simulink model "pendulum_project"  (Simulink 4.00)
settings: Solver=ode45  SolverMode=SingleTasking  StartTime=0.0  StopTime=100  RelTol=1e-4  AbsTol=1e-7
libraries: simulink3 x1
settings Model: LimitDataPoints=off  BlockReductionOpt=off

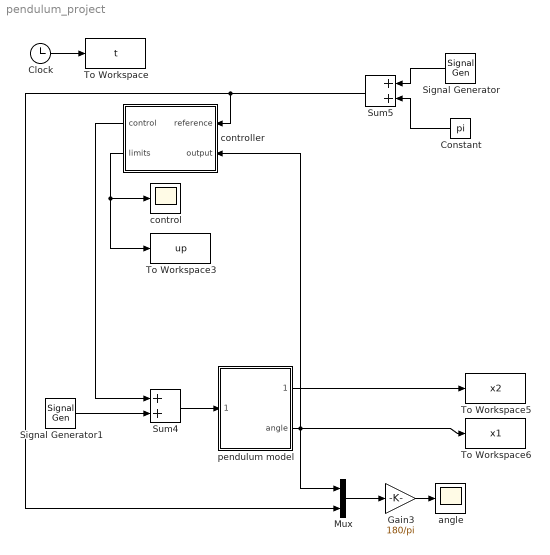
== system pendulum_project ==
  Clock : Clock
      settings: DisplayTime=off  Decimation=10
  Constant : Constant  Orientation=left  Value=pi
  Gain3 : Gain  Gain=180/pi  Multiplication=Element-wise(K.*u)  SaturateOnIntegerOverflow=on
  Mux : Mux  Inputs=2
  Signal Generator : SignalGenerator  Orientation=left  WaveForm=square  Amplitude=12*pi/180  Frequency=.1  Units=Hertz
  Signal Generator1 : SignalGenerator  WaveForm=square  Amplitude=.1  Frequency=.04  Units=Hertz
  Sum4 : Sum  Inputs=++  SaturateOnIntegerOverflow=on
  Sum5 : Sum  Orientation=left  Inputs=++  SaturateOnIntegerOverflow=on
  To Workspace : ToWorkspace  VariableName=t  SampleTime=.01  SaveFormat=Array
  To Workspace3 : ToWorkspace  VariableName=up  SampleTime=.01  SaveFormat=Array
  To Workspace5 : ToWorkspace  VariableName=x2  SampleTime=.01  SaveFormat=Array
  To Workspace6 : ToWorkspace  VariableName=x1  SampleTime=.01  SaveFormat=Array
  angle : Scope
      settings: TickLabels=on  TimeRange=100  YMin=165  YMax=195  SaveToWorkspace=off  SaveName=ScopeData  DataFormat=Array  MaxDataPoints=10000
  control : Scope
      settings: TickLabels=on  TimeRange=100  YMin=-2  YMax=2  SaveToWorkspace=off  SaveName=ScopeData  DataFormat=Array  MaxDataPoints=10000
  controller : Subsystem  Orientation=left
      settings: RTWFcnNameOpts=Auto  RTWFileNameOpts=Auto
  pendulum model : Subsystem  mask{mass=.275, length=0.5, friction=.01, Tmax=.5, quant=.1, stiction=.01, IC=0}
      mask prompts: friction "friction coeff"; Tmax "Max Torque"; quant "quantization (deg)"; stiction "stiction dead-zone (rad/s)"; IC "Initial condition (deg, 0 velocity)"
      settings: RTWFcnNameOpts=Auto  RTWFileNameOpts=Auto
  wires:
  pendulum model/1(velocity) -> To Workspace5/1
  Sum4/1 -> pendulum model/1(control)
  Signal Generator1/1 -> Sum4/2
  Gain3/1 -> angle/1
  Clock/1 -> To Workspace/1
  controller/1(control) -> Sum4/1
  controller/2(limits) -> control/1, To Workspace3/1
  pendulum model/2(angle) -> To Workspace6/1, Mux/1, controller/2(output)
  Signal Generator/1 -> Sum5/1
  Constant/1 -> Sum5/2
  Sum5/1 -> controller/1(reference), Mux/2
  Mux/1 -> Gain3/1

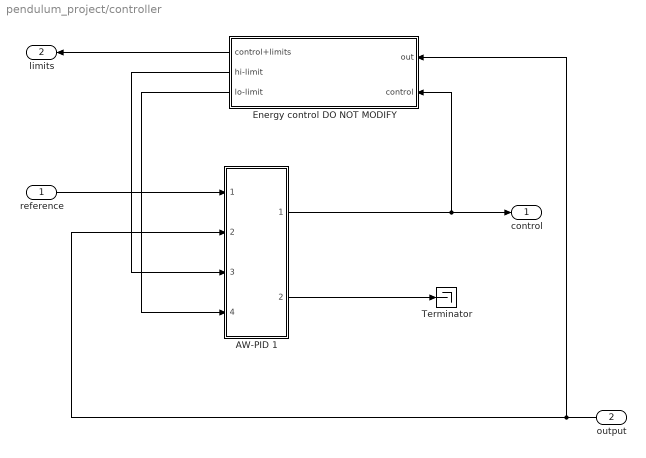
== system pendulum_project/controller ==
  reference : Inport  Port=1  LatchInput=off
  output : Inport  Orientation=left  Port=2  LatchInput=off
  AW-PID 1 : Subsystem  mask(Anti-windup PID ){kpid=[11, 30, 1.5], TCD=.01, TF=0, DT=.01, ipole=0, t_pref=[0.05, 0.4]}
      mask prompts: kpid "PID parameters [kp,ki,kd]"; TCD "Pseudo-derivative filter time constant"; TF "Error lowpass filter Time constant"; DT "Sampling Time"; ipole "Approx. Integrator pole"; t_pref "Reference prefilter [num,den] time constants"
      mask help: Discrete PID with Anti-windup, prefilter, and lowpass filter
      mask init:
      | t_z=t_pref(1);t_p=t_pref(2);
      settings: RTWFcnNameOpts=Auto  RTWFileNameOpts=Auto
      mask Display: disp('AW-PID\n+filter+init')
  Energy control DO NOT MODIFY : Subsystem  Orientation=left
      settings: RTWFcnNameOpts=Auto  RTWFileNameOpts=Auto
  Terminator : Terminator
  control : Outport  Port=1  InitialOutput=0
  limits : Outport  Orientation=left  Port=2  InitialOutput=0
  wires:
  Energy control DO NOT MODIFY/1(control+limits) -> limits/1
  output/1 -> Energy control DO NOT MODIFY/1(out), AW-PID 1/2(System Output)
  AW-PID 1/2(sat_indicator) -> Terminator/1
  AW-PID 1/1(Input to system) -> control/1, Energy control DO NOT MODIFY/2(control)
  reference/1 -> AW-PID 1/1(Set point)
  Energy control DO NOT MODIFY/2(hi-limit) -> AW-PID 1/3(input constraint hi)
  Energy control DO NOT MODIFY/3(lo-limit) -> AW-PID 1/4(input constraint lo)

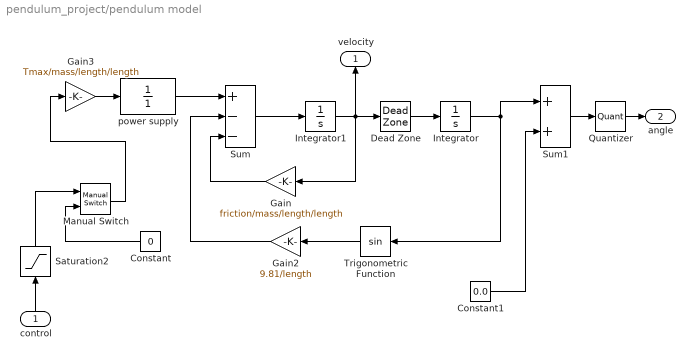
== system pendulum_project/pendulum model ==
  control : Inport  Orientation=up  Port=1  LatchInput=off
  Constant : Constant  Orientation=left  Value=0
  Constant1 : Constant  Value=0.0
  Dead Zone : DeadZone  LowerValue=-stiction  UpperValue=stiction  SaturateOnIntegerOverflow=on  LinearizeAsGain=on
  Gain : Gain  Orientation=left  Gain=friction/mass/length/length  Multiplication=Element-wise(K.*u)  SaturateOnIntegerOverflow=on
  Gain2 : Gain  Orientation=left  Gain=9.81/length  Multiplication=Element-wise(K.*u)  SaturateOnIntegerOverflow=on
  Gain3 : Gain  Gain=Tmax/mass/length/length  Multiplication=Element-wise(K.*u)  SaturateOnIntegerOverflow=on
  Integrator : Integrator  ExternalReset=none  InitialConditionSource=internal  InitialCondition=IC*pi/180  LimitOutput=off  UpperSaturationLimit=inf  LowerSaturationLimit=-inf  ShowSaturationPort=off  ShowStatePort=off  AbsoluteTolerance=auto
  Integrator1 : Integrator  ExternalReset=none  InitialConditionSource=internal  InitialCondition=0  LimitOutput=off  UpperSaturationLimit=inf  LowerSaturationLimit=-inf  ShowSaturationPort=off  ShowStatePort=off  AbsoluteTolerance=auto
  Manual Switch : simulink3/Nonlinear/Manual Switch  sw=1  action=0
  Quantizer : Quantizer  QuantizationInterval=quant*pi/180  LinearizeAsGain=on
  Saturation2 : Saturate  Orientation=up  UpperLimit=1  LowerLimit=-1  LinearizeAsGain=on
  Sum : Sum  Inputs=+--  SaturateOnIntegerOverflow=on
  Sum1 : Sum  Inputs=++  SaturateOnIntegerOverflow=on
  Trigonometric Function : Trigonometry  Orientation=left  Operator=sin  OutputSignalType=auto
  power supply : TransferFcn  Numerator=1  Denominator=1  AbsoluteTolerance=auto  Realization=auto
  velocity : Outport  Orientation=up  Port=1  InitialOutput=0
  angle : Outport  Port=2  InitialOutput=0
  wires:
  Sum/1 -> Integrator1/1
  Integrator1/1 -> Gain/1, velocity/1, Dead Zone/1
  Gain/1 -> Sum/3
  Dead Zone/1 -> Integrator/1
  Integrator/1 -> Sum1/1, Trigonometric Function/1
  Trigonometric Function/1 -> Gain2/1
  Gain2/1 -> Sum/2
  Gain3/1 -> power supply/1
  power supply/1 -> Sum/1
  control/1 -> Saturation2/1
  Manual Switch/1 -> Gain3/1
  Constant/1 -> Manual Switch/2
  Constant1/1 -> Sum1/2
  Sum1/1 -> Quantizer/1
  Quantizer/1 -> angle/1
  Saturation2/1 -> Manual Switch/1

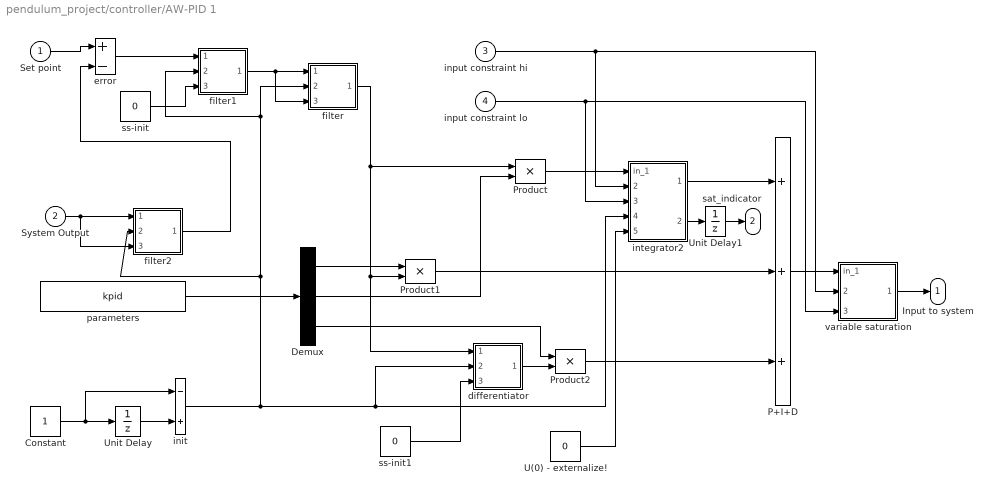
== system pendulum_project/controller/AW-PID 1 ==
  Set point : Inport  Port=1  LatchInput=off
  System Output : Inport  Port=2  LatchInput=off
  input constraint hi : Inport  Port=3  LatchInput=off
  input constraint lo : Inport  Port=4  LatchInput=off
  Constant : Constant  Value=1
  Demux : Demux  Outputs=3  BusSelectionMode=off
  P+I+D : Sum  Inputs=+++  SaturateOnIntegerOverflow=on
  Product : Product  Inputs=2  Multiplication=Element-wise(.*)  SaturateOnIntegerOverflow=on
  Product1 : Product  Inputs=2  Multiplication=Element-wise(.*)  SaturateOnIntegerOverflow=on
  Product2 : Product  Inputs=2  Multiplication=Element-wise(.*)  SaturateOnIntegerOverflow=on
  U(0) - externalize! : Constant  Value=0
  Unit Delay : UnitDelay  X0=0  SampleTime=DT
      settings: RTWStateStorageClass=Auto
  Unit Delay1 : UnitDelay  X0=0  SampleTime=DT
      settings: RTWStateStorageClass=Auto
  differentiator : Subsystem  mask(Approx. Differentator){DT=DT, TC=TCD}
      mask prompts: DT "sampling time"; TC "Time constant"
      settings: RTWFcnNameOpts=Auto  RTWFileNameOpts=Auto
  error : Sum  Inputs=+-  SaturateOnIntegerOverflow=on
  filter : Subsystem  mask(Lead-Lag Filter){DT=DT, TC=TF, TZ=0}
      mask prompts: DT "sampling time"; TC "Pole Time constant"; TZ "Zero Time Constant"
      settings: RTWFcnNameOpts=Auto  RTWFileNameOpts=Auto
  filter1 : Subsystem  mask(Lead-Lag Filter){DT=DT, TC=t_p, TZ=t_z}
      mask prompts: DT "sampling time"; TC "Pole Time constant"; TZ "Zero Time Constant"
      settings: RTWFcnNameOpts=Auto  RTWFileNameOpts=Auto
  filter2 : Subsystem  mask(Lead-Lag Filter){DT=DT, TC=t_z, TZ=t_p}
      mask prompts: DT "sampling time"; TC "Pole Time constant"; TZ "Zero Time Constant"
      settings: RTWFcnNameOpts=Auto  RTWFileNameOpts=Auto
  init : Sum  Inputs=-+  SaturateOnIntegerOverflow=on
  integrator2 : Subsystem  mask(Anti windup intgrator){DT=DT, pole=ipole}
      mask prompts: DT "sampling time"
      mask help: Integral with anti-windup
      settings: RTWFcnNameOpts=Auto  RTWFileNameOpts=Auto
  parameters : Constant  Value=kpid
  ss-init : Constant  Value=0
  ss-init1 : Constant  Value=0
  variable saturation : Subsystem  mask(Anti windup intgrator){DT=DT}
      mask prompts: DT "sampling time"
      mask help: Integral with anti-windup
      settings: RTWFcnNameOpts=Auto  RTWFileNameOpts=Auto
      mask Display: disp('DT-I-AW')
  Input to system : Outport  Port=1  InitialOutput=0
  sat_indicator : Outport  Port=2  InitialOutput=0
  wires:
  input constraint hi/1 -> variable saturation/2(umax), integrator2/2(umax)
  input constraint lo/1 -> variable saturation/3(umin), integrator2/3(umin)
  variable saturation/1(out_1) -> Input to system/1
  filter2/1(out_1) -> error/2
  System Output/1 -> filter2/1(in_1), filter2/3(init val)
  filter1/1(out_1) -> filter/1(in_1), filter/3(init val)
  Product2/1 -> P+I+D/3
  Demux/2 -> Product/2
  Demux/1 -> Product1/1
  Product/1 -> integrator2/1(in_1)
  P+I+D/1 -> variable saturation/1(in_1)
  integrator2/1(out_1) -> P+I+D/1
  error/1 -> filter1/1(in_1)
  parameters/1 -> Demux/1
  Set point/1 -> error/1
  Product1/1 -> P+I+D/2
  Demux/3 -> Product2/1
  differentiator/1(out_1) -> Product2/2
  filter/1(out_1) -> Product/1, Product1/2, differentiator/1(in_1)
  Constant/1 -> Unit Delay/1, init/1
  Unit Delay/1 -> init/2
  init/1 -> differentiator/2(init flag), integrator2/4(init flag), filter2/2(init flag), filter/2(init flag), filter1/2(init flag)
  integrator2/2(out_2) -> Unit Delay1/1
  U(0) - externalize!/1 -> integrator2/5(init val)
  ss-init/1 -> filter1/3(init val)
  ss-init1/1 -> differentiator/3(init val)
  Unit Delay1/1 -> sat_indicator/1

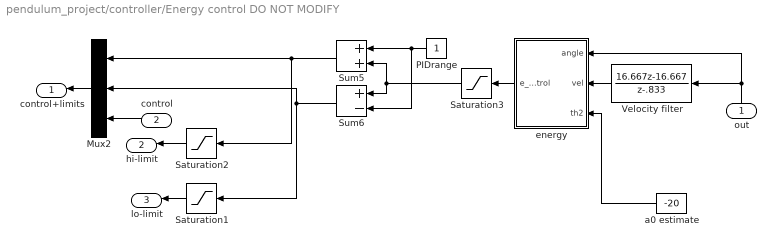
== system pendulum_project/controller/Energy control DO NOT MODIFY ==
  out : Inport  Orientation=up  Port=1  LatchInput=off
  control : Inport  Orientation=left  Port=2  LatchInput=off
  Mux2 : Mux  Orientation=left  Inputs=3
      settings: DisplayOption=none
  PIDrange : Constant  Orientation=left  Value=1
  Saturation1 : Saturate  Orientation=left  UpperLimit=1  LowerLimit=-1  LinearizeAsGain=on
  Saturation2 : Saturate  Orientation=left  UpperLimit=1  LowerLimit=-1  LinearizeAsGain=on
  Saturation3 : Saturate  Orientation=left  UpperLimit=1  LowerLimit=-1  LinearizeAsGain=on
  Sum5 : Sum  Orientation=left  Inputs=++  SaturateOnIntegerOverflow=on
  Sum6 : Sum  Orientation=left  Inputs=+-  SaturateOnIntegerOverflow=on
  Velocity filter : DiscreteTransferFcn  Orientation=left  Numerator="[16.667  -16.667]"  Denominator=[1 -.833]  SampleTime=.01  Realization=auto
      settings: RTWStateStorageClass=Auto
  a0 estimate : Constant  Orientation=left  Value=-20
  energy : Subsystem  Orientation=left
      settings: RTWFcnNameOpts=Auto  RTWFileNameOpts=Auto
  control+limits : Outport  Orientation=left  Port=1
  hi-limit : Outport  Orientation=left  Port=2
  lo-limit : Outport  Orientation=left  Port=3
  wires:
  Sum5/1 -> Mux2/1, Saturation2/1
  Sum6/1 -> Mux2/2, Saturation1/1
  energy/1(e_control) -> Saturation3/1
  Velocity filter/1 -> energy/2(vel)
  PIDrange/1 -> Sum5/1, Sum6/2
  Saturation3/1 -> Sum6/1, Sum5/2
  out/1 -> Velocity filter/1, energy/1(angle)
  a0 estimate/1 -> energy/3(th2)
  control/1 -> Mux2/3
  Mux2/1 -> control+limits/1
  Saturation2/1 -> hi-limit/1
  Saturation1/1 -> lo-limit/1

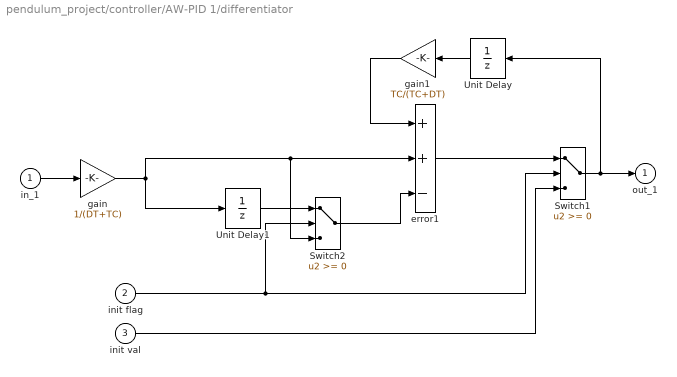
== system pendulum_project/controller/AW-PID 1/differentiator ==
  in_1 : Inport  Port=1  LatchInput=off
  init flag : Inport  Port=2  LatchInput=off
  init val : Inport  Port=3  LatchInput=off
  Switch1 : Switch  Threshold=0
  Switch2 : Switch  Threshold=0
  Unit Delay : UnitDelay  Orientation=left  X0=0  SampleTime=DT
      settings: RTWStateStorageClass=Auto
  Unit Delay1 : UnitDelay  X0=0  SampleTime=DT
      settings: RTWStateStorageClass=Auto
  error1 : Sum  Inputs=++-  SaturateOnIntegerOverflow=on
  gain : Gain  Gain=1/(DT+TC)  Multiplication=Element-wise(K.*u)  SaturateOnIntegerOverflow=on
  gain1 : Gain  Orientation=left  Gain=TC/(TC+DT)  Multiplication=Element-wise(K.*u)  SaturateOnIntegerOverflow=on
  out_1 : Outport  Port=1  InitialOutput=0
  wires:
  init val/1 -> Switch1/3
  init flag/1 -> Switch1/2, Switch2/2
  error1/1 -> Switch1/1
  Switch1/1 -> out_1/1, Unit Delay/1
  in_1/1 -> gain/1
  gain/1 -> Unit Delay1/1, Switch2/3, error1/2
  Unit Delay/1 -> gain1/1
  Unit Delay1/1 -> Switch2/1
  Switch2/1 -> error1/3
  gain1/1 -> error1/1

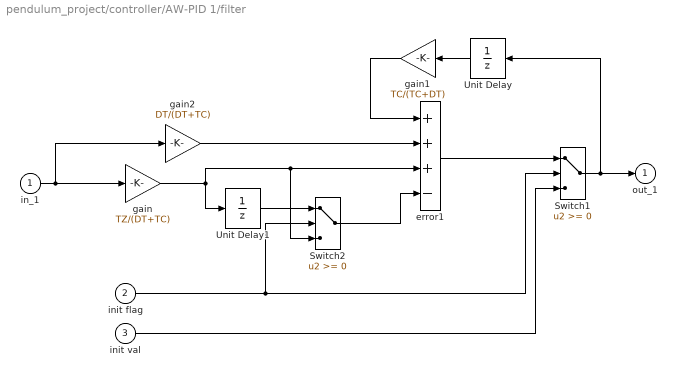
== system pendulum_project/controller/AW-PID 1/filter ==
  in_1 : Inport  Port=1  LatchInput=off
  init flag : Inport  Port=2  LatchInput=off
  init val : Inport  Port=3  LatchInput=off
  Switch1 : Switch  Threshold=0
  Switch2 : Switch  Threshold=0
  Unit Delay : UnitDelay  Orientation=left  X0=0  SampleTime=DT
      settings: RTWStateStorageClass=Auto
  Unit Delay1 : UnitDelay  X0=0  SampleTime=DT
      settings: RTWStateStorageClass=Auto
  error1 : Sum  Inputs=+++-  SaturateOnIntegerOverflow=on
  gain : Gain  Gain=TZ/(DT+TC)  Multiplication=Element-wise(K.*u)  SaturateOnIntegerOverflow=on
  gain1 : Gain  Orientation=left  Gain=TC/(TC+DT)  Multiplication=Element-wise(K.*u)  SaturateOnIntegerOverflow=on
  gain2 : Gain  Gain=DT/(DT+TC)  Multiplication=Element-wise(K.*u)  SaturateOnIntegerOverflow=on
  out_1 : Outport  Port=1  InitialOutput=0
  wires:
  gain1/1 -> error1/1
  Switch2/1 -> error1/4
  Unit Delay1/1 -> Switch2/1
  Unit Delay/1 -> gain1/1
  gain/1 -> error1/3, Switch2/3, Unit Delay1/1
  in_1/1 -> gain/1, gain2/1
  Switch1/1 -> Unit Delay/1, out_1/1
  error1/1 -> Switch1/1
  init flag/1 -> Switch2/2, Switch1/2
  init val/1 -> Switch1/3
  gain2/1 -> error1/2

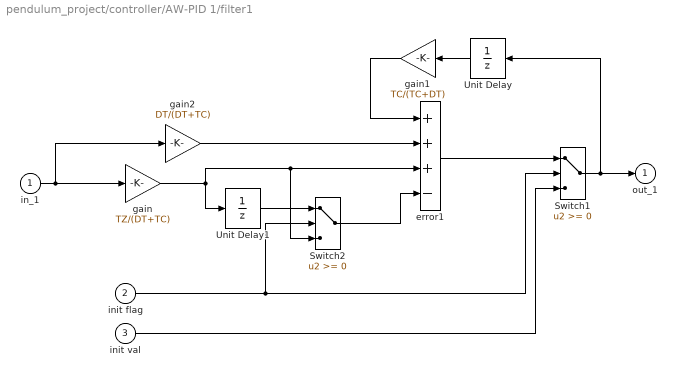
== system pendulum_project/controller/AW-PID 1/filter1 ==
  in_1 : Inport  Port=1  LatchInput=off
  init flag : Inport  Port=2  LatchInput=off
  init val : Inport  Port=3  LatchInput=off
  Switch1 : Switch  Threshold=0
  Switch2 : Switch  Threshold=0
  Unit Delay : UnitDelay  Orientation=left  X0=0  SampleTime=DT
      settings: RTWStateStorageClass=Auto
  Unit Delay1 : UnitDelay  X0=0  SampleTime=DT
      settings: RTWStateStorageClass=Auto
  error1 : Sum  Inputs=+++-  SaturateOnIntegerOverflow=on
  gain : Gain  Gain=TZ/(DT+TC)  Multiplication=Element-wise(K.*u)  SaturateOnIntegerOverflow=on
  gain1 : Gain  Orientation=left  Gain=TC/(TC+DT)  Multiplication=Element-wise(K.*u)  SaturateOnIntegerOverflow=on
  gain2 : Gain  Gain=DT/(DT+TC)  Multiplication=Element-wise(K.*u)  SaturateOnIntegerOverflow=on
  out_1 : Outport  Port=1  InitialOutput=0
  wires:
  gain2/1 -> error1/2
  init val/1 -> Switch1/3
  init flag/1 -> Switch1/2, Switch2/2
  error1/1 -> Switch1/1
  Switch1/1 -> out_1/1, Unit Delay/1
  in_1/1 -> gain2/1, gain/1
  gain/1 -> Unit Delay1/1, Switch2/3, error1/3
  Unit Delay/1 -> gain1/1
  Unit Delay1/1 -> Switch2/1
  Switch2/1 -> error1/4
  gain1/1 -> error1/1

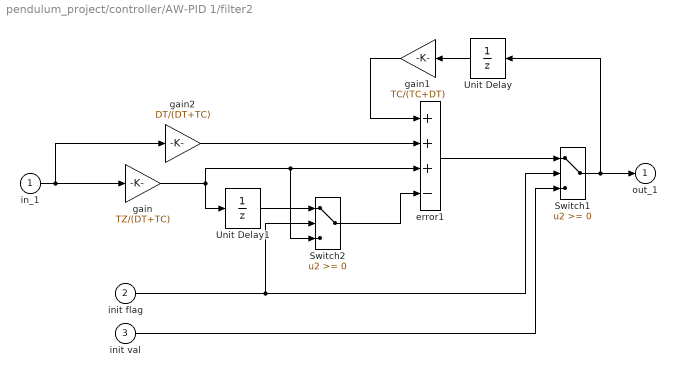
== system pendulum_project/controller/AW-PID 1/filter2 ==
  in_1 : Inport  Port=1  LatchInput=off
  init flag : Inport  Port=2  LatchInput=off
  init val : Inport  Port=3  LatchInput=off
  Switch1 : Switch  Threshold=0
  Switch2 : Switch  Threshold=0
  Unit Delay : UnitDelay  Orientation=left  X0=0  SampleTime=DT
      settings: RTWStateStorageClass=Auto
  Unit Delay1 : UnitDelay  X0=0  SampleTime=DT
      settings: RTWStateStorageClass=Auto
  error1 : Sum  Inputs=+++-  SaturateOnIntegerOverflow=on
  gain : Gain  Gain=TZ/(DT+TC)  Multiplication=Element-wise(K.*u)  SaturateOnIntegerOverflow=on
  gain1 : Gain  Orientation=left  Gain=TC/(TC+DT)  Multiplication=Element-wise(K.*u)  SaturateOnIntegerOverflow=on
  gain2 : Gain  Gain=DT/(DT+TC)  Multiplication=Element-wise(K.*u)  SaturateOnIntegerOverflow=on
  out_1 : Outport  Port=1  InitialOutput=0
  wires:
  gain1/1 -> error1/1
  Switch2/1 -> error1/4
  Unit Delay1/1 -> Switch2/1
  Unit Delay/1 -> gain1/1
  gain/1 -> error1/3, Switch2/3, Unit Delay1/1
  in_1/1 -> gain/1, gain2/1
  Switch1/1 -> Unit Delay/1, out_1/1
  error1/1 -> Switch1/1
  init flag/1 -> Switch2/2, Switch1/2
  init val/1 -> Switch1/3
  gain2/1 -> error1/2

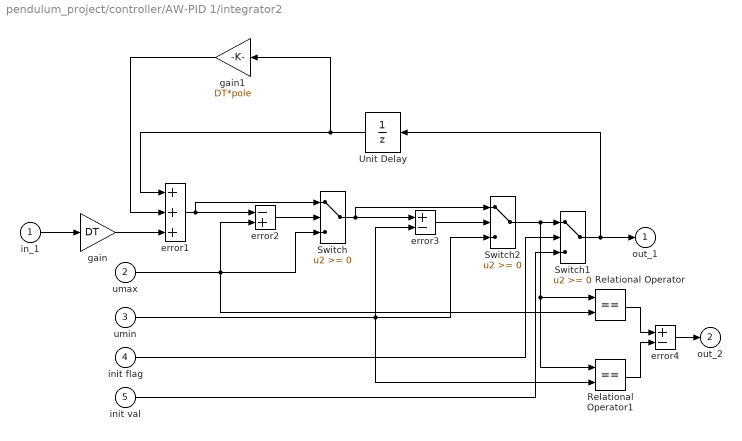
== system pendulum_project/controller/AW-PID 1/integrator2 ==
  in_1 : Inport  Port=1  LatchInput=off
  umax : Inport  Port=2  LatchInput=off
  umin : Inport  Port=3  LatchInput=off
  init flag : Inport  Port=4  LatchInput=off
  init val : Inport  Port=5  LatchInput=off
  Relational Operator : RelationalOperator  Operator===
  Relational Operator1 : RelationalOperator  Operator===
  Switch : Switch  Threshold=0
  Switch1 : Switch  Threshold=0
  Switch2 : Switch  Threshold=0
  Unit Delay : UnitDelay  Orientation=left  X0=0  SampleTime=DT
      settings: RTWStateStorageClass=Auto
  error1 : Sum  Inputs=+++  SaturateOnIntegerOverflow=on
  error2 : Sum  Inputs=-+  SaturateOnIntegerOverflow=on
  error3 : Sum  Inputs=+-  SaturateOnIntegerOverflow=on
  error4 : Sum  Inputs=+-  SaturateOnIntegerOverflow=on
  gain : Gain  Gain=DT  Multiplication=Element-wise(K.*u)  SaturateOnIntegerOverflow=on
  gain1 : Gain  Orientation=left  Gain=DT*pole  Multiplication=Element-wise(K.*u)  SaturateOnIntegerOverflow=on
  out_1 : Outport  Port=1  InitialOutput=0
  out_2 : Outport  Port=2  InitialOutput=0
  wires:
  in_1/1 -> gain/1
  error1/1 -> Switch/1, error2/1
  umax/1 -> Switch/3, error2/2, Relational Operator/2
  umin/1 -> Switch2/3, error3/2, Relational Operator1/2
  error3/1 -> Switch2/2
  error2/1 -> Switch/2
  gain/1 -> error1/3
  gain1/1 -> error1/2
  Switch1/1 -> out_1/1, Unit Delay/1
  Switch2/1 -> Switch1/1, Relational Operator/1, Relational Operator1/1
  init flag/1 -> Switch1/2
  init val/1 -> Switch1/3
  Switch/1 -> error3/1, Switch2/1
  Relational Operator1/1 -> error4/2
  Relational Operator/1 -> error4/1
  error4/1 -> out_2/1
  Unit Delay/1 -> error1/1, gain1/1

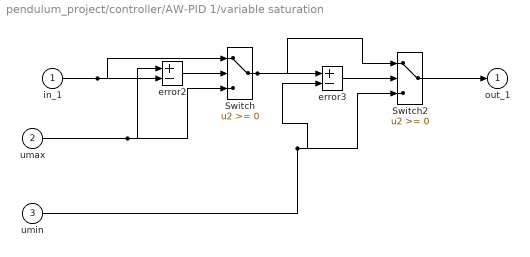
== system pendulum_project/controller/AW-PID 1/variable saturation ==
  in_1 : Inport  Port=1  LatchInput=off
  umax : Inport  Port=2  LatchInput=off
  umin : Inport  Port=3  LatchInput=off
  Switch : Switch  Threshold=0
  Switch2 : Switch  Threshold=0
  error2 : Sum  Inputs=+-  SaturateOnIntegerOverflow=on
  error3 : Sum  Inputs=+-  SaturateOnIntegerOverflow=on
  out_1 : Outport  Port=1  InitialOutput=0
  wires:
  error2/1 -> Switch/2
  error3/1 -> Switch2/2
  umin/1 -> error3/2, Switch2/3
  umax/1 -> error2/1, Switch/3
  Switch/1 -> error3/1, Switch2/1
  Switch2/1 -> out_1/1
  in_1/1 -> error2/2, Switch/1

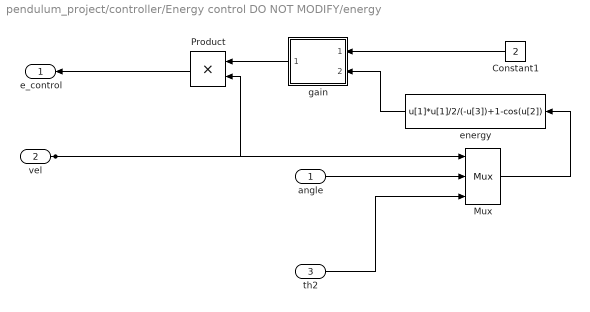
== system pendulum_project/controller/Energy control DO NOT MODIFY/energy ==
  angle : Inport  Port=1  LatchInput=off
  vel : Inport  Port=2  LatchInput=off
  th2 : Inport  Port=3  LatchInput=off
  Constant1 : Constant  Orientation=left  Value=2
  Mux : Mux  Inputs=3
      settings: DisplayOption=none
  Product : Product  Orientation=left  Inputs=2  Multiplication=Element-wise(.*)  SaturateOnIntegerOverflow=on
  energy : Fcn  Orientation=left  Expr=u[1]*u[1]/2/(-u[3])+1-cos(u[2])
  gain : Subsystem  Orientation=left  mask{kp=20, edz=.05}
      mask prompts: kp "Gain"; edz "error dead-zone limits"
      mask help: Discrete PID with Anti-windup and with lowpass filter
      settings: RTWFcnNameOpts=Auto  RTWFileNameOpts=Auto
  e_control : Outport  Orientation=left  Port=1
  wires:
  vel/1 -> Mux/1, Product/2
  th2/1 -> Mux/3
  angle/1 -> Mux/2
  gain/1(Input to system) -> Product/1
  energy/1 -> gain/2(System Output)
  Constant1/1 -> gain/1(Set point)
  Product/1 -> e_control/1
  Mux/1 -> energy/1

== system pendulum_project/controller/Energy control DO NOT MODIFY/energy/gain ==
  Set point : Inport  Port=1  LatchInput=off
  System Output : Inport  Port=2  LatchInput=off
  Fcn : Fcn  Expr=u[1]*u[1]*u[1]/(edz*edz+u[1]*u[1])
  Proportional : Gain  Gain=kp  Multiplication=Element-wise(K.*u)  SaturateOnIntegerOverflow=on
  error : Sum  Inputs=+-  SaturateOnIntegerOverflow=on
  Input to system : Outport  Port=1  InitialOutput=0
  wires:
  Fcn/1 -> Proportional/1
  error/1 -> Fcn/1
  System Output/1 -> error/2
  Set point/1 -> error/1
  Proportional/1 -> Input to system/1
